simulink model "mod3_2plus1MASH_v2"  (Simulink 7.9)
settings: Solver=VariableStepDiscrete  StartTime=0.0  StopTime=simu.trantime  RelTol=1e-3
undefined symbols (not defined in the file or in its folder): dfilt, Fs, mod
libraries: dspsigops x4, dspsrcs4 x2, dsparch4 x1
settings Model: Creator=amyles  LastModifiedBy=Arnaldi Isacco
settings DataIOCC: MaxDataPoints=50000
settings OptimizationCC: InlineParams=on
settings DebuggingCC: StrictBusMsg=Warning
settings ModelReferenceCC: ModelReferenceNumInstancesAllowed=Single
settings CodeAppCC: CustomSymbolStrType=$N$R$M_T
settings GRTTargetCC: CombineOutputUpdateFcns=off  GRTInterface=on

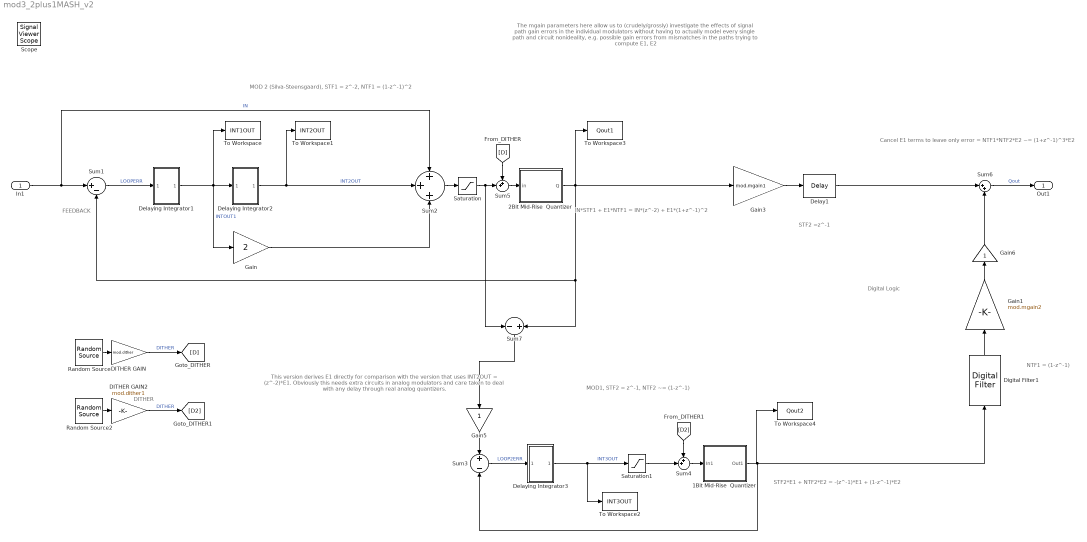
== system mod3_2plus1MASH_v2 ==
  note: MOD 2 (Silva-Steensgaard), STF1 = z^-2, NTF1 = (1-z^-1)^2
  note: MOD1, STF2 = z^-1, NTF2 ~= (1-z^-1)
  note: IN*STF1 + E1*NTF1 =
      | IN*(z^-2) + E1*(1+z^-1)^2
  note: STF2*E1 + NTF2*E2
      | = -(z^-1)*E1 + (1-z^-1)*E2
  note: Cancel E1 terms to leave only
      |
      | error = NTF1*NTF2*E2
      | ~= (1+z^-1)^3*E2
  note: DITHER
  note: FEEDBACK
  note: Digital Logic
  note: NTF1 = (1-z^-1)
  note: The mgain parameters here allow us to (crudely/grossly) investigate the effects of signal path gain
      | errors in the individual modulators without having to actually model every single path and
      | circuit nonideality, e.g. possible gain errors from mismatches in the paths trying to compute E1, E2
  note: This version derives E1
      | directly for comparison
      | with the version that uses
      | INT2OUT = (z^-2)*E1.
      | Obviously this needs extra
      | circuits in analog modulators
      | and care taken to deal with
      | any delay through real
      | analog quantizers.
  note: STF2
      | =z^-1
  In1 : Inport
  1Bit Mid-Rise  Quantizer : Subsystem
  2Bit Mid-Rise  Quantizer : Subsystem
  DITHER GAIN : Gain  Gain=mod.dither  SampleTime=1/Fs
  DITHER GAIN2 : Gain  Gain=mod.dither1  SampleTime=1/Fs
  Delay1 : dspsigops/Delay  InputProcessing=Inherited (this choice will be removed - see release notes)  dly_unit=Samples  delay=1  ic_detail=off  dif_ic_for_ch=off  dif_ic_for_dly=off  ic=0  reset_popup=None
  Delaying Integrator1 : Subsystem
  Delaying Integrator2 : Subsystem
  Delaying Integrator3 : Subsystem
  Digital Filter1 : dsparch4/Digital Filter  TypePopup=FIR (all zeros)  IIRFiltStruct=Direct form II transposed  AllPoleFiltStruct=Direct form  FIRFiltStruct=Direct form  CoeffSource=Specify via dialog  NumCoeffs=[1 -2 1]  DenCoeffs=[1 0.1]  BiQuadCoeffs=[1 0.3 0.4 1 0.1 0.2]  LatticeCoeffs=[0.2 0.4]  denIgnore=on  FiltPerSampPopup=One filter per frame  IC=0  ICnum=0  ICden=0  roundingMode=Floor  overflowMode=off  ScaleValues=1  scaleValueFracLength=14  stageInFracLength=15  stageOutFracLength=15  FilterSource=Specify via dialog  dfiltObjectName=dfilt.dffir([1 2 1])  InputProcessing=Inherited (this choice will be removed - see release notes)
  Gain : Gain  Gain=2
  Gain1 : Gain  Gain=mod.mgain2
  Gain3 : Gain  Gain=mod.mgain1
  Gain5 : Gain
      settings: AttributesFormatString=Option to scale input\nfor saturation control...
  Gain6 : Gain
      settings: AttributesFormatString=Option to un-scale input\npost saturation control...
  Random Source : dspsrcs4/Random Source  SrcType=Uniform  NormMethod=Ziggurat  CltLength=12  MinVal=-1  MaxVal=1  MeanVal=0  VarVal=1  RepMode=Not repeatable  rawSeed=1  IsInherit=off  SampMode=Discrete  SampTime=1/Fs  SampFrame=1  DataType=Double  OutComplex=Real
  Random Source2 : dspsrcs4/Random Source  SrcType=Uniform  NormMethod=Ziggurat  CltLength=12  MinVal=-1  MaxVal=1  MeanVal=0  VarVal=1  RepMode=Not repeatable  rawSeed=1  IsInherit=off  SampMode=Discrete  SampTime=1/Fs  SampFrame=1  DataType=Double  OutComplex=Real
  Saturation : Saturate  UpperLimit=mod.qsatin1  LowerLimit=-(mod.qsatin1)
  Saturation1 : Saturate  UpperLimit=mod.qsatin2  LowerLimit=-(mod.qsatin2)
  Sum1 : Sum  Inputs=|+-  SampleTime=1/Fs
  Sum2 : Sum  Inputs=+++
  Sum3 : Sum  Inputs=+-
  Sum4 : Sum  Inputs=++|
  Sum5 : Sum  Inputs=++|
  Sum6 : Sum  Inputs=|++
  Sum7 : Sum  Inputs=-+
  To Workspace : ToWorkspace  VariableName=INT1OUT  SampleTime=-1
  To Workspace1 : ToWorkspace  VariableName=INT2OUT  SampleTime=-1
  To Workspace2 : ToWorkspace  VariableName=INT3OUT  SampleTime=-1
  To Workspace3 : ToWorkspace  VariableName=Qout1  SampleTime=-1
  To Workspace4 : ToWorkspace  VariableName=Qout2  SampleTime=-1
  Out1 : Outport
  Scope : SignalViewerScope  IOType=viewer  NumInputPorts=4  ZoomMode=xonly  RefreshTime=0.035000
      settings: YMin=-5~-5~-5~-5  YMax=5~5~5~5
  wires:
  Sum1/1 -> Delaying Integrator1/1(In1)  "LOOPERR"
  In1/1 -> Sum1/1, Sum2/1  "IN"
  Gain/1 -> Sum2/3
  Delaying Integrator2/1(Out1) -> To Workspace1/1, Sum2/2  "INT2OUT"
  Sum3/1 -> Delaying Integrator3/1(In1)  "LOOP2ERR"
  Delaying Integrator1/1(Out1) -> Gain/1, To Workspace/1, Delaying Integrator2/1(In1)  "INTOUT1"
  Sum2/1 -> Saturation/1
  Delaying Integrator3/1(Out1) -> Saturation1/1, To Workspace2/1  "INT3OUT"
  1Bit Mid-Rise  Quantizer/1(Out1) -> Sum3/2, To Workspace4/1, Digital Filter1/1
  Gain1/1 -> Gain6/1
  Sum6/1 -> Out1/1  "Qout"
  Digital Filter1/1 -> Gain1/1
  Gain6/1 -> Sum6/2
  2Bit Mid-Rise  Quantizer/1(Q) -> Gain3/1, To Workspace3/1, Sum1/2, Sum7/2
  Saturation1/1 -> Sum4/2
  Gain3/1 -> Delay1/1
  Random Source/1 -> DITHER GAIN/1
  DITHER GAIN/1 -> [D]  "DITHER"
  Random Source2/1 -> DITHER GAIN2/1
  DITHER GAIN2/1 -> [D2]  "DITHER"
  Saturation/1 -> Sum5/2, Sum7/1
  [D] -> Sum5/1
  Sum5/1 -> 2Bit Mid-Rise  Quantizer/1(in)
  [D2] -> Sum4/1
  Sum4/1 -> 1Bit Mid-Rise  Quantizer/1(In1)
  Sum7/1 -> Gain5/1
  Gain5/1 -> Sum3/1
  Delay1/1 -> Sum6/1

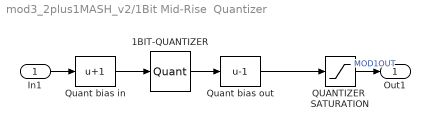
== system mod3_2plus1MASH_v2/1Bit Mid-Rise  Quantizer ==
  In1 : Inport
  1BIT-QUANTIZER : Quantizer  QuantizationInterval=2  LinearizeAsGain=off  SampleTime=1/Fs
      settings: AttributesFormatString=step = 2
  QUANTIZER  SATURATION : Saturate  UpperLimit=mod.qsatout2  LowerLimit=-(mod.qsatout2)
      settings: AttributesFormatString=Limit quantizer\noutput
  Quant bias in : Bias  Bias=1
      settings: AttributesFormatString=Need offset to give\nMID-RISE quantiser
  Quant bias out : Bias  Bias=-1
      settings: AttributesFormatString=Shift outputs to\n..., -2, 1, 1, ...
  Out1 : Outport
  wires:
  Quant bias out/1 -> QUANTIZER  SATURATION/1
  Quant bias in/1 -> 1BIT-QUANTIZER/1
  1BIT-QUANTIZER/1 -> Quant bias out/1
  QUANTIZER  SATURATION/1 -> Out1/1  "MOD1OUT"
  In1/1 -> Quant bias in/1

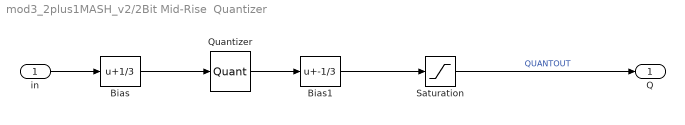
== system mod3_2plus1MASH_v2/2Bit Mid-Rise  Quantizer ==
  in : Inport
  Bias : Bias  Bias=1/3
      settings: AttributesFormatString=Need offset to give\nMID-RISE quantiser
  Bias1 : Bias  Bias=-1/3
  Quantizer : Quantizer  QuantizationInterval=2/3  LinearizeAsGain=off  SampleTime=1/Fs
  Saturation : Saturate  UpperLimit=mod.qsatout1  LowerLimit=-(mod.qsatout1)
  Q : Outport
  wires:
  Bias/1 -> Quantizer/1
  Saturation/1 -> Q/1  "QUANTOUT"
  Quantizer/1 -> Bias1/1
  Bias1/1 -> Saturation/1
  in/1 -> Bias/1

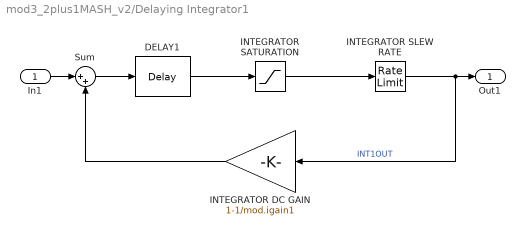
== system mod3_2plus1MASH_v2/Delaying Integrator1 ==
  In1 : Inport
  DELAY1 : dspsigops/Delay  InputProcessing=Inherited (this choice will be removed - see release notes)  dly_unit=Samples  delay=1  ic_detail=off  dif_ic_for_ch=off  dif_ic_for_dly=off  ic=0  reset_popup=None
  INTEGRATOR SATURATION : Saturate  UpperLimit=mod.isat1  LowerLimit=-(mod.isat1)
      settings: AttributesFormatString=Real integrators will have\noutput swing limits (analog\nsignal headroom or digital\naccumulator min/max values)
  INTEGRATOR SLEW RATE : RateLimiter  RisingSlewLimit=mod.isr1  FallingSlewLimit=-(mod.isr1)  SampleTimeMode=inherited
      settings: AttributesFormatString=...and\nmay suffer from\npoor slew rate
  INTEGRATOR DC GAIN : Gain  Gain=1-1/mod.igain1
      settings: AttributesFormatString=Integrator leakage\n(model finite integrator dc/LF\ngain in analog modulators)
  Sum : Sum  Inputs=|++
      settings: AttributesFormatString=Integrator\nsummer
  Out1 : Outport
  wires:
  Sum/1 -> DELAY1/1
  INTEGRATOR DC GAIN/1 -> Sum/2
  INTEGRATOR SLEW RATE/1 -> INTEGRATOR DC GAIN/1, Out1/1  "INT1OUT"
  INTEGRATOR SATURATION/1 -> INTEGRATOR SLEW RATE/1
  In1/1 -> Sum/1
  DELAY1/1 -> INTEGRATOR SATURATION/1

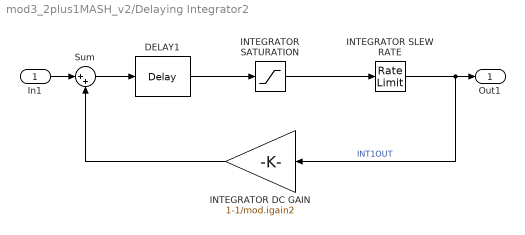
== system mod3_2plus1MASH_v2/Delaying Integrator2 ==
  In1 : Inport
  DELAY1 : dspsigops/Delay  InputProcessing=Inherited (this choice will be removed - see release notes)  dly_unit=Samples  delay=1  ic_detail=off  dif_ic_for_ch=off  dif_ic_for_dly=off  ic=0  reset_popup=None
  INTEGRATOR SATURATION : Saturate  UpperLimit=mod.isat2  LowerLimit=-(mod.isat2)
      settings: AttributesFormatString=Real integrators will have\noutput swing limits (analog\nsignal headroom or digital\naccumulator min/max values)
  INTEGRATOR SLEW RATE : RateLimiter  RisingSlewLimit=mod.isr2  FallingSlewLimit=-(mod.isr2)  SampleTimeMode=inherited
      settings: AttributesFormatString=...and\nmay suffer from\npoor slew rate
  INTEGRATOR DC GAIN : Gain  Gain=1-1/mod.igain2
      settings: AttributesFormatString=Integrator leakage\n(model finite integrator dc/LF\ngain in analog modulators)
  Sum : Sum  Inputs=|++
      settings: AttributesFormatString=Integrator\nsummer
  Out1 : Outport
  wires:
  Sum/1 -> DELAY1/1
  INTEGRATOR DC GAIN/1 -> Sum/2
  INTEGRATOR SLEW RATE/1 -> INTEGRATOR DC GAIN/1, Out1/1  "INT1OUT"
  INTEGRATOR SATURATION/1 -> INTEGRATOR SLEW RATE/1
  In1/1 -> Sum/1
  DELAY1/1 -> INTEGRATOR SATURATION/1

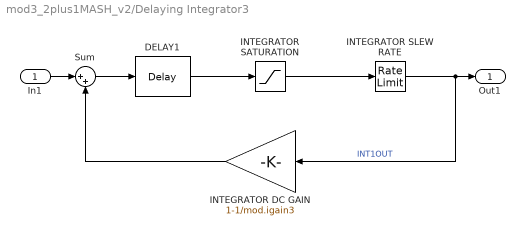
== system mod3_2plus1MASH_v2/Delaying Integrator3 ==
  In1 : Inport
  DELAY1 : dspsigops/Delay  InputProcessing=Inherited (this choice will be removed - see release notes)  dly_unit=Samples  delay=1  ic_detail=off  dif_ic_for_ch=off  dif_ic_for_dly=off  ic=0  reset_popup=None
  INTEGRATOR SATURATION : Saturate  UpperLimit=mod.isat3  LowerLimit=-(mod.isat3)
      settings: AttributesFormatString=Real integrators will have\noutput swing limits (analog\nsignal headroom or digital\naccumulator min/max values)
  INTEGRATOR SLEW RATE : RateLimiter  RisingSlewLimit=mod.isr3  FallingSlewLimit=-(mod.isr3)  SampleTimeMode=inherited
      settings: AttributesFormatString=...and\nmay suffer from\npoor slew rate
  INTEGRATOR DC GAIN : Gain  Gain=1-1/mod.igain3
      settings: AttributesFormatString=Integrator leakage\n(model finite integrator dc/LF\ngain in analog modulators)
  Sum : Sum  Inputs=|++
      settings: AttributesFormatString=Integrator\nsummer
  Out1 : Outport
  wires:
  Sum/1 -> DELAY1/1
  INTEGRATOR DC GAIN/1 -> Sum/2
  INTEGRATOR SLEW RATE/1 -> INTEGRATOR DC GAIN/1, Out1/1  "INT1OUT"
  INTEGRATOR SATURATION/1 -> INTEGRATOR SLEW RATE/1
  In1/1 -> Sum/1
  DELAY1/1 -> INTEGRATOR SATURATION/1
